simulink model "control_pid_sim"  (R2023b)
settings: Solver=VariableStepAuto  StartTime=0.0  StopTime=50  RelTol=1e-3
values from neighbouring files (symbols this model uses):
  kd = 0.00013    [control_pid.m]
  ki = 0.6    [control_pid.m]
  kp = 1.3    [control_pid.m]
  ref = 0.1    [control_pid.m]
libraries: cstblocks x1
settings Model: Creator=Lucas  LastModifiedBy=Lucas

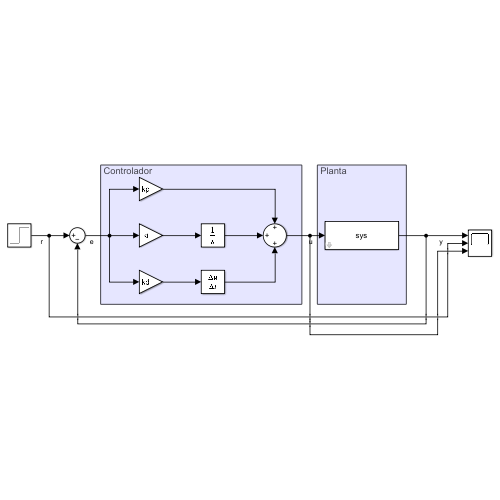
[thumbnail: Simulink's stored preview of the top-level diagram]
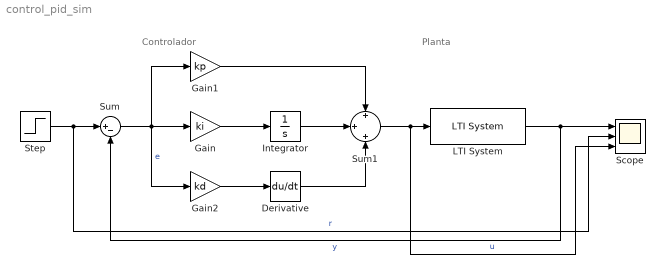
== system control_pid_sim ==
  note: Controlador
  note: Planta
  Derivative : Derivative
  Gain : Gain  Gain=ki
  Gain1 : Gain  Gain=kp
  Gain2 : Gain  Gain=kd
  Integrator : Integrator
  LTI System : cstblocks/LTI System  sys=sys  IC=[]  PadeOrder=0
  Scope : Scope  NumInputPorts=3
  Step : Step  After=ref  SampleTime=0
  Sum : Sum  Inputs=|+-
  Sum1 : Sum  Inputs=+|+|+
  wires:
  Step/1 -> Scope/2, Sum/1  "r"
  Gain/1 -> Integrator/1
  Gain2/1 -> Derivative/1
  Integrator/1 -> Sum1/2
  Gain1/1 -> Sum1/1
  Derivative/1 -> Sum1/3
  Sum/1 -> Gain2/1, Gain1/1, Gain/1  "e"
  Sum1/1 -> Scope/3, LTI System/1  "u"
  LTI System/1 -> Sum/2, Scope/1  "y"
